simulink model "Thruster"  (R2019b)
settings: Solver=VariableStepAuto  StartTime=0.0  StopTime=10.0  RelTol=1e-3
values from neighbouring files (symbols this model uses):
  Jm = 4.0e-6    (= 4e-06)    [parameters.m]
  km = 0.042    [parameters.m]
  kt = 0.042    [parameters.m]
  Lm = 1.16/1000    (= 0.00116)    [parameters.m]
  Rm = 8.4    [parameters.m]
undefined symbols (not defined in the file or in its folder): B_friction, K_aero
settings Model: Creator=peter  LastModifiedBy=peter

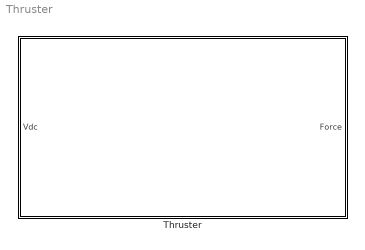
== system Thruster ==
  Thruster : Subsystem

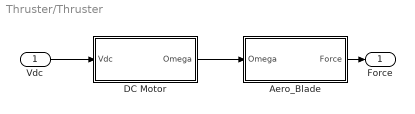
== system Thruster/Thruster ==
  Vdc : Inport
  Aero_Blade : Subsystem
  "DC Motor " : Subsystem
  Force : Outport
  wires:
  Aero_Blade/1(Force) -> Force/1
  Vdc/1 -> "DC Motor "/1(Vdc)
  "DC Motor "/1(Omega) -> Aero_Blade/1(Omega)

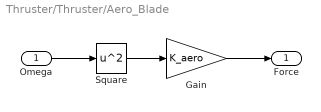
== system Thruster/Thruster/Aero_Blade ==
  Omega : Inport
  Gain : Gain  Gain=K_aero
  Square : Math  Operator=square  SignedPower=off  SaturateOnIntegerOverflow=on
  Force : Outport
  wires:
  Omega/1 -> Square/1
  Gain/1 -> Force/1
  Square/1 -> Gain/1

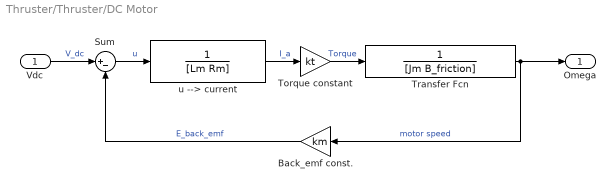
== system Thruster/Thruster/DC Motor  ==
  Vdc : Inport
  Back_emf const. : Gain  Gain=km
  Sum : Sum  Inputs=|+-
  Torque constant : Gain  Gain=kt
  Transfer Fcn : TransferFcn  Denominator=[Jm B_friction]
  u --> current : TransferFcn  Denominator=[Lm Rm]
  Omega : Outport
  wires:
  Sum/1 -> u --> current/1  "u"
  u --> current/1 -> Torque constant/1  "I_a"
  Vdc/1 -> Sum/1  "V_dc"
  Back_emf const./1 -> Sum/2  "E_back_emf"
  Torque constant/1 -> Transfer Fcn/1  "Torque"
  Transfer Fcn/1 -> Back_emf const./1, Omega/1  "motor speed"
